simulink model "BergmanInOut_incomplet"  (R2025b)
settings: Solver=VariableStepAuto  StartTime=0.0  StopTime=200  RelTol=1e-3
values from neighbouring files (symbols this model uses):
  Gb = 92    [Dev_04_M.m]
  Ib = 7.3    [Dev_04_M.m]
  n = 0.3    [Dev_04_M.m]
  p1 = 0.03    [Dev_04_M.m]
  p2 = 0.02    [Dev_04_M.m]
  p3 = 1.06*(10^-5)    (= 1.06e-05)    [Dev_04_M.m]
  x0 = [92; 0; 7.3; 0]    [Dev_04_M.m]
settings Model: Creator=casie  LastModifiedBy=Louis

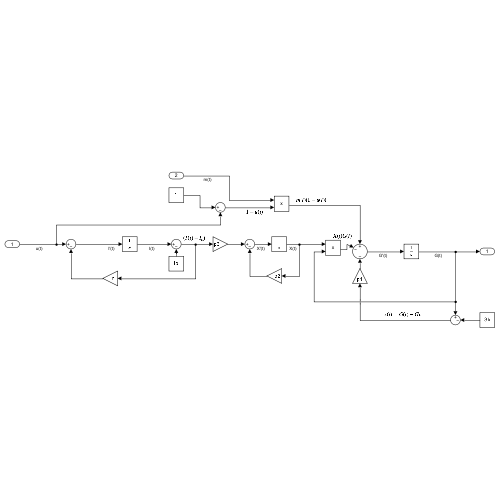
[thumbnail: Simulink's stored preview of the top-level diagram]
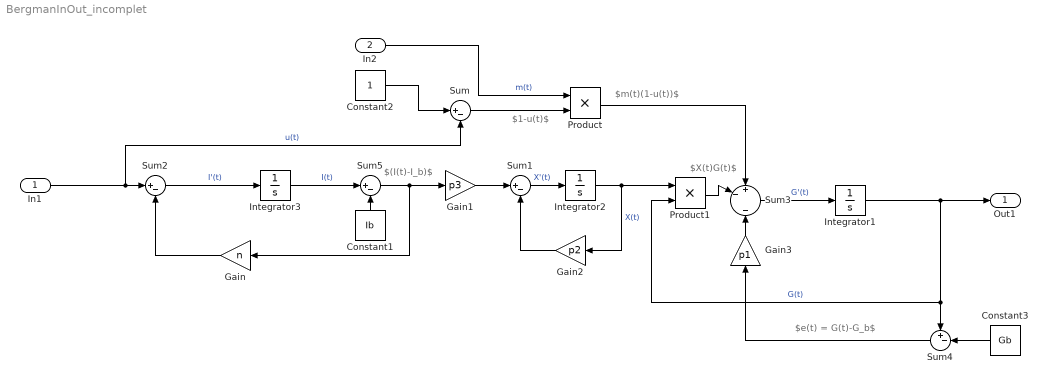
== system BergmanInOut_incomplet ==
  note: $X(t)G(t)$
  note: $e(t) = G(t)-G_b$
  note: $m(t)(1-u(t))$
  note: $1-u(t)$
  note: $(I(t)-I_b)$
  In1 : Inport
  In2 : Inport  Port=2
  Constant1 : Constant  Value=Ib
  Constant2 : Constant
  Constant3 : Constant  Value=Gb
  Gain : Gain  Gain=n
  Gain1 : Gain  Gain=p3
  Gain2 : Gain  Gain=p2
  Gain3 : Gain  Gain=p1
  Integrator1 : Integrator  InitialCondition=x0(1)
  Integrator2 : Integrator  InitialCondition=x0(2)
  Integrator3 : Integrator  InitialCondition=x0(3)
  Product : Product
  Product1 : Product
  Sum{,1..2,5} (4 alike) : Sum  Inputs=|+-
  Sum3 : Sum  Inputs=+-|-
  Sum4 : Sum  Inputs=+-|
  Out1 : Outport
  wires:
  In2/1 -> Product/1  "m(t)"
  Sum3/1 -> Integrator1/1  "G'(t)"
  Sum1/1 -> Integrator2/1  "X'(t)"
  In1/1 -> Sum2/1, Sum/2  "u(t)"
  Integrator3/1 -> Sum5/1  "I(t)"
  Integrator1/1 -> Sum4/1, Product1/2, Out1/1  "G(t)"
  Sum2/1 -> Integrator3/1  "I'(t)"
  Integrator2/1 -> Product1/1, Gain2/1  "X(t)"
  Sum4/1 -> Gain3/1
  Constant3/1 -> Sum4/2
  Gain/1 -> Sum2/2
  Constant1/1 -> Sum5/2
  Sum5/1 -> Gain/1, Gain1/1
  Gain1/1 -> Sum1/1
  Gain2/1 -> Sum1/2
  Constant2/1 -> Sum/1
  Sum/1 -> Product/2
  Product/1 -> Sum3/1
  Gain3/1 -> Sum3/3
  Product1/1 -> Sum3/2
